simulink model "CP_SFC_NLin_n9558292"  (R2018a)
settings: Solver=ode4  StartTime=0.0  StopTime=5  FixedStep=0.02  RelTol=1e-3
values from neighbouring files (symbols this model uses):
  g = 9.81    [CP_SFC_Lin_a_MainFile_n9558292.m]
  K_SF = Ka    [CP_SFC_Lin_a_MainFile_n9558292.m]
  l = 0.2    [CP_SFC_Lin_a_MainFile_n9558292.m]
  m = 0.15    [CP_SFC_Lin_a_MainFile_n9558292.m]
  Mc = 0.4    [CP_SFC_Lin_a_MainFile_n9558292.m]
  x10 = 0.2    [CP_SFC_Lin_a_MainFile_n9558292.m]
  x20 = deg2rad(20)    [CP_SFC_Lin_a_MainFile_n9558292.m]
  x2_bar = 0    [CP_SFC_Lin_a_MainFile_n9558292.m]
  x30 = 0    [CP_SFC_Lin_a_MainFile_n9558292.m]
  x40 = 0    [CP_SFC_Lin_a_MainFile_n9558292.m]
settings Model: Creator=haidarobeid  LastModifiedBy=haidarobeid

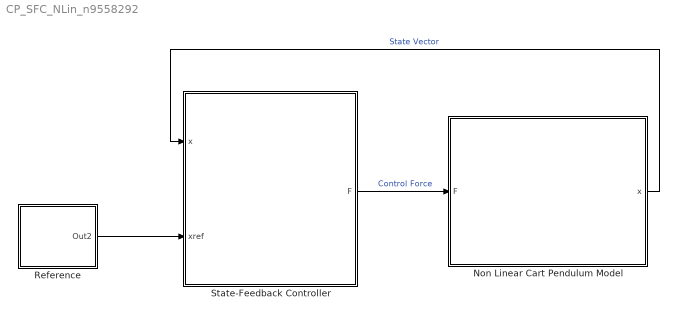
== system CP_SFC_NLin_n9558292 ==
  Non Linear Cart Pendulum Model : Subsystem
  Reference : Subsystem
  State-Feedback Controller : Subsystem
  wires:
  State-Feedback Controller/1("F ") -> Non Linear Cart Pendulum Model/1(F)  "Control Force"
  Non Linear Cart Pendulum Model/1(x) -> State-Feedback Controller/1(x)  "State Vector"
  Reference/1(Out2) -> State-Feedback Controller/2(xref)

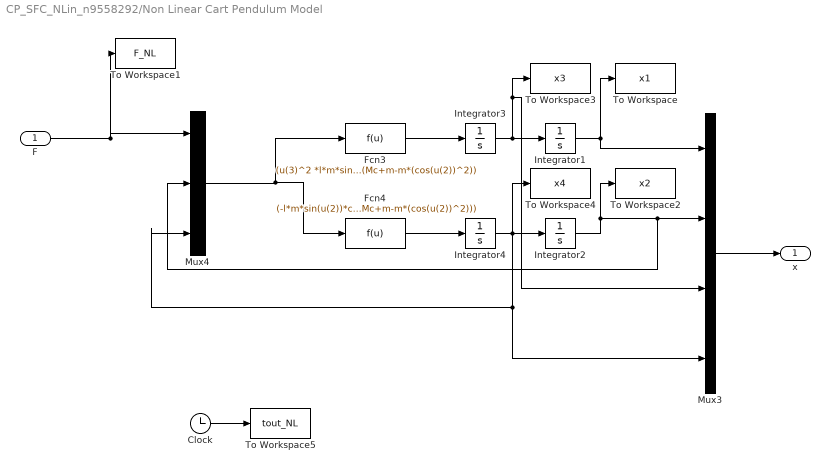
== system CP_SFC_NLin_n9558292/Non Linear Cart Pendulum Model ==
  F : Inport
  Clock : Clock
  Fcn3 : Fcn  Expr=(u(3)^2 *l*m*sin(u(2)) - g*m*sin(u(2))*cos(u(2)) +u(1))/(Mc+m-m*(cos(u(2))^2))
  Fcn4 : Fcn  Expr=(-l*m*sin(u(2))*cos(u(2))*u(3)^2 + g*(Mc+m)*sin(u(2)) - cos(u(2))*u(1) )/(l*(Mc+m-m*(cos(u(2))^2)))
  Integrator1 : Integrator  InitialCondition=x10
  Integrator2 : Integrator  InitialCondition=x20
  Integrator3 : Integrator  InitialCondition=x30
  Integrator4 : Integrator  InitialCondition=x40
  Mux3 : Mux
  Mux4 : Mux  Inputs=3
  To Workspace : ToWorkspace  VariableName=x1  SampleTime=-1
  To Workspace1 : ToWorkspace  VariableName=F_NL  SampleTime=-1
  To Workspace2 : ToWorkspace  VariableName=x2  SampleTime=-1
  To Workspace3 : ToWorkspace  VariableName=x3  SampleTime=-1
  To Workspace4 : ToWorkspace  VariableName=x4  SampleTime=-1
  To Workspace5 : ToWorkspace  VariableName=tout_NL  SampleTime=-1
  x : Outport
  wires:
  Fcn3/1 -> Integrator3/1
  Fcn4/1 -> Integrator4/1
  Mux3/1 -> x/1
  Integrator4/1 -> Mux4/3, Mux3/4, Integrator2/1, To Workspace4/1
  Integrator2/1 -> To Workspace2/1, Mux4/2, Mux3/2
  F/1 -> To Workspace1/1, Mux4/1
  Integrator1/1 -> Mux3/1, To Workspace/1
  Integrator3/1 -> Integrator1/1, Mux3/3, To Workspace3/1
  Mux4/1 -> Fcn4/1, Fcn3/1
  Clock/1 -> To Workspace5/1

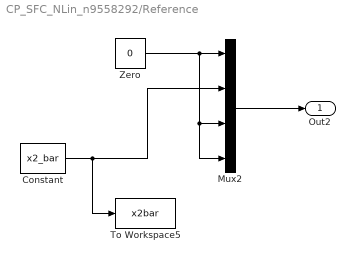
== system CP_SFC_NLin_n9558292/Reference ==
  Constant : Constant  Value=x2_bar
  Mux2 : Mux
  To Workspace5 : ToWorkspace  VariableName=x2bar  SaveFormat=Timeseries  SampleTime=-1
  Zero : Constant  Value=0
  Out2 : Outport
  wires:
  Mux2/1 -> Out2/1
  Constant/1 -> To Workspace5/1, Mux2/2
  Zero/1 -> Mux2/4, Mux2/3, Mux2/1

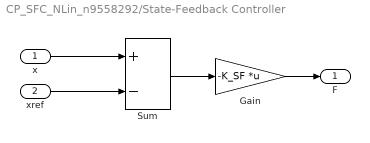
== system CP_SFC_NLin_n9558292/State-Feedback Controller ==
  x : Inport
  xref : Inport  Port=2
  Gain : Gain  Gain=-K_SF  Multiplication=Matrix(K*u)
  Sum : Sum  Inputs=+-
  "F " : Outport
  wires:
  xref/1 -> Sum/2
  Gain/1 -> "F "/1
  x/1 -> Sum/1
  Sum/1 -> Gain/1
